simulink model "ourCar"  (R2017a)
settings: Solver=VariableStepAuto  StartTime=0.0  StopTime=15  RelTol=1e-3
undefined symbols (not defined in the file): l, L, magnitude
libraries: simulink x2
settings Model: Creator=Erebus  LastModifiedBy=Sno0ker
settings SolverCC: MaxConsecutiveMinStep=25  AlgebraicLoopSolver=LineSearch

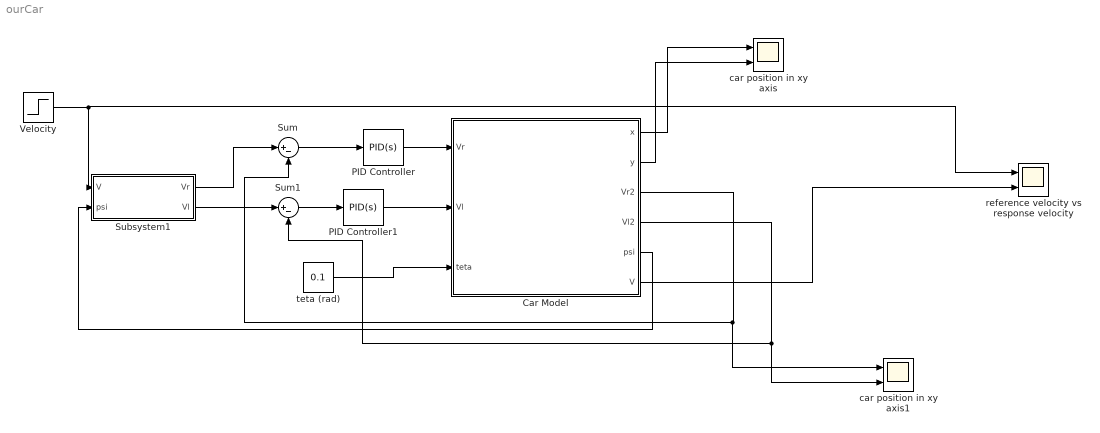
== system ourCar ==
  Car Model : Subsystem
  PID Controller : simulink/Continuous/PID Controller  Controller=PID  TimeDomain=Continuous-time  SampleTime=-1  IntegratorMethod=Forward Euler  FilterMethod=Forward Euler  Form=Parallel  UseFilter=on  ControllerParametersSource=internal  P=1.2  I=1  D=0  N=100  InitialConditionSource=internal  InitialConditionForIntegrator=0  InitialConditionForFilter=0  ExternalReset=none  LimitOutput=off  UpperSaturationLimit=inf  LowerSaturationLimit=-inf  LinearizeAsGain=on  AntiWindupMode=none  Kb=1  TrackingMode=off  Kt=1  PParamMin=[]  PParamMax=[]  IParamMin=[]  IParamMax=[]  DParamMin=[]  DParamMax=[]  NParamMin=[]  NParamMax=[]  KbParamMin=[]  KbParamMax=[]  KtParamMin=[]  KtParamMax=[]  POutMin=[]  POutMax=[]  IOutMin=[]  IOutMax=[]  DOutMin=[]  DOutMax=[]  NOutMin=[]  NOutMax=[]  KbOutMin=[]  KbOutMax=[]  KtOutMin=[]  KtOutMax=[]  IntegratorOutMin=[]  IntegratorOutMax=[]  FilterOutMin=[]  FilterOutMax=[]  SumOutMin=[]  SumOutMax=[]  SumI1OutMin=[]  SumI1OutMax=[]  SumI2OutMin=[]  SumI2OutMax=[]  SumI3OutMin=[]  SumI3OutMax=[]  SumDOutMin=[]  SumDOutMax=[]  SaturationOutMin=[]  SaturationOutMax=[]  IntegratorContinuousStateAttributes=''  IntegratorStateMustResolveToSignalObject=off  IntegratorRTWStateStorageClass=Auto  FilterContinuousStateAttributes=''  FilterStateMustResolveToSignalObject=off  FilterRTWStateStorageClass=Auto  DifferentiatorICPrevScaledInput=0  DifferentiatorOutMin=[]  DifferentiatorOutMax=[]  InitialConditionSetting=State (most efficient)
  PID Controller1 : simulink/Continuous/PID Controller  Controller=PID  TimeDomain=Continuous-time  SampleTime=-1  IntegratorMethod=Forward Euler  FilterMethod=Forward Euler  Form=Parallel  UseFilter=on  ControllerParametersSource=internal  P=1  I=1  D=0  N=100  InitialConditionSource=internal  InitialConditionForIntegrator=0  InitialConditionForFilter=0  ExternalReset=none  LimitOutput=off  UpperSaturationLimit=inf  LowerSaturationLimit=-inf  LinearizeAsGain=on  AntiWindupMode=none  Kb=1  TrackingMode=off  Kt=1  PParamMin=[]  PParamMax=[]  IParamMin=[]  IParamMax=[]  DParamMin=[]  DParamMax=[]  NParamMin=[]  NParamMax=[]  KbParamMin=[]  KbParamMax=[]  KtParamMin=[]  KtParamMax=[]  POutMin=[]  POutMax=[]  IOutMin=[]  IOutMax=[]  DOutMin=[]  DOutMax=[]  NOutMin=[]  NOutMax=[]  KbOutMin=[]  KbOutMax=[]  KtOutMin=[]  KtOutMax=[]  IntegratorOutMin=[]  IntegratorOutMax=[]  FilterOutMin=[]  FilterOutMax=[]  SumOutMin=[]  SumOutMax=[]  SumI1OutMin=[]  SumI1OutMax=[]  SumI2OutMin=[]  SumI2OutMax=[]  SumI3OutMin=[]  SumI3OutMax=[]  SumDOutMin=[]  SumDOutMax=[]  SaturationOutMin=[]  SaturationOutMax=[]  IntegratorContinuousStateAttributes=''  IntegratorStateMustResolveToSignalObject=off  IntegratorRTWStateStorageClass=Auto  FilterContinuousStateAttributes=''  FilterStateMustResolveToSignalObject=off  FilterRTWStateStorageClass=Auto  DifferentiatorICPrevScaledInput=0  DifferentiatorOutMin=[]  DifferentiatorOutMax=[]  InitialConditionSetting=State (most efficient)
  Subsystem1 : Subsystem
  Sum : Sum  Inputs=|+-
  Sum1 : Sum  Inputs=|+-
  "Velocity " : Step  SampleTime=0
  car position in xy axis : Scope  NumInputPorts=2
  car position in xy axis1 : Scope  NumInputPorts=2
  reference velocity vs response velocity : Scope  NumInputPorts=2
  teta (rad) : Constant  Value=0.1
  wires:
  Car Model/1(x) -> car position in xy axis/1
  Car Model/2(y) -> car position in xy axis/2
  "Velocity "/1 -> reference velocity vs response velocity/1, Subsystem1/1(V)
  teta (rad)/1 -> Car Model/3(teta)
  Car Model/5(psi) -> Subsystem1/2(psi)
  Subsystem1/1(Vr) -> Sum/1
  Subsystem1/2(Vl) -> Sum1/1
  Car Model/4("Vl2 ") -> car position in xy axis1/2, Sum1/2
  Sum/1 -> PID Controller/1
  PID Controller/1 -> Car Model/1(Vr)
  Sum1/1 -> PID Controller1/1
  PID Controller1/1 -> Car Model/2("Vl ")
  Car Model/6(V) -> reference velocity vs response velocity/2
  Car Model/3(Vr2) -> car position in xy axis1/1, Sum/2

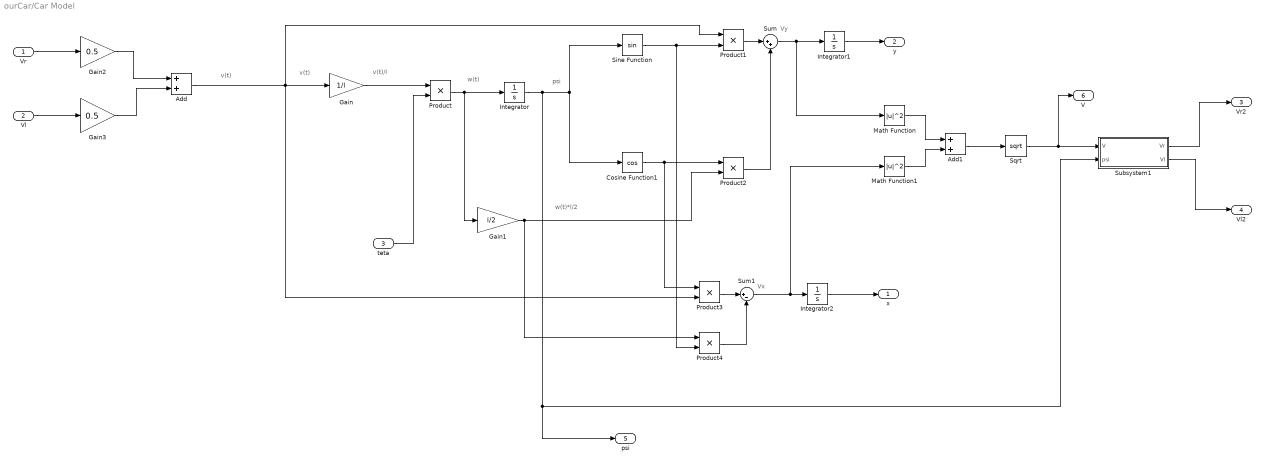
== system ourCar/Car Model ==
  note: v(t)
  note: w(t)*l/2
  note: v(t)/l
  note: v(t)
  note: Vy
  note: psi
  note: Vx
  note: w(t)
  Vr : Inport
  "Vl " : Inport  Port=2
  teta : Inport  Port=3
  Add : Sum
  Add1 : Sum
  Cosine Function1 : Trigonometry  Operator=cos
  Gain : Gain  Gain=1/l
  Gain1 : Gain  Gain=l/2
  Gain2 : Gain  Gain=0.5
  Gain3 : Gain  Gain=0.5
  Integrator : Integrator
  Integrator1 : Integrator
  Integrator2 : Integrator
  Math Function : Math  Operator=magnitude^2  SaturateOnIntegerOverflow=on
  Math Function1 : Math  Operator=magnitude^2  SaturateOnIntegerOverflow=on
  Product{,1..4} (5 alike) : Product
  Sine Function : Trigonometry
  Sqrt : Sqrt  SaturateOnIntegerOverflow=on
  Subsystem1 : Subsystem
  Sum : Sum  Inputs=|++
  Sum1 : Sum  Inputs=|+-
  x : Outport
  y : Outport  Port=2
  Vr2 : Outport  Port=3
  "Vl2 " : Outport  Port=4
  psi : Outport  Port=5
  V : Outport  Port=6
  wires:
  Product/1 -> Gain1/1, Integrator/1
  Product3/1 -> Sum1/1
  Sum1/1 -> Math Function1/1, Integrator2/1
  teta/1 -> Product/2
  Integrator1/1 -> y/1
  Product2/1 -> Sum/2
  Product1/1 -> Sum/1
  Gain/1 -> Product/1
  Gain1/1 -> Product2/2, Product4/1
  Sum/1 -> Math Function/1, Integrator1/1
  Product4/1 -> Sum1/2
  Sine Function/1 -> Product4/2, Product1/2
  Cosine Function1/1 -> Product2/1, Product3/1
  Add/1 -> Product3/2, Product1/1, Gain/1
  Integrator2/1 -> x/1
  Vr/1 -> Gain2/1
  "Vl "/1 -> Gain3/1
  Gain2/1 -> Add/1
  Gain3/1 -> Add/2
  Math Function/1 -> Add1/1
  Math Function1/1 -> Add1/2
  Add1/1 -> Sqrt/1
  Integrator/1 -> Subsystem1/2(psi), psi/1, Cosine Function1/1, Sine Function/1
  Subsystem1/1(Vr) -> Vr2/1
  Subsystem1/2(Vl) -> "Vl2 "/1
  Sqrt/1 -> V/1, Subsystem1/1(V)

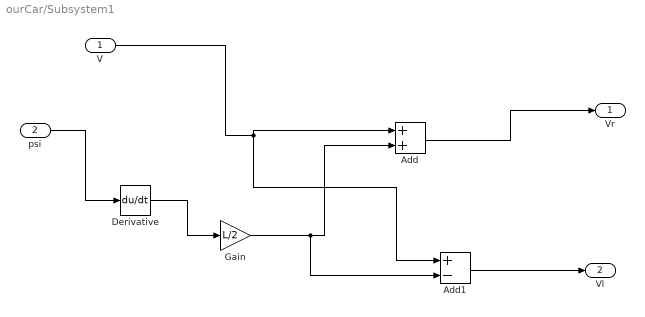
== system ourCar/Subsystem1 ==
  V : Inport
  psi : Inport  Port=2
  Add : Sum
  Add1 : Sum  Inputs=+-
  Derivative : Derivative
  Gain : Gain  Gain=L/2
  Vr : Outport
  Vl : Outport  Port=2
  wires:
  V/1 -> Add1/1, Add/1
  Gain/1 -> Add1/2, Add/2
  Add/1 -> Vr/1
  Add1/1 -> Vl/1
  psi/1 -> Derivative/1
  Derivative/1 -> Gain/1

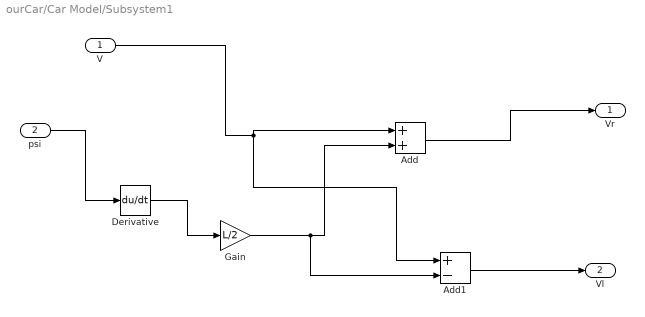
== system ourCar/Car Model/Subsystem1 ==
  V : Inport
  psi : Inport  Port=2
  Add : Sum
  Add1 : Sum  Inputs=+-
  Derivative : Derivative
  Gain : Gain  Gain=L/2
  Vr : Outport
  Vl : Outport  Port=2
  wires:
  V/1 -> Add1/1, Add/1
  Gain/1 -> Add1/2, Add/2
  Add/1 -> Vr/1
  Add1/1 -> Vl/1
  psi/1 -> Derivative/1
  Derivative/1 -> Gain/1
